simulink model "QPSK_Rayleigh_Channel"  (R2023b)
settings: Solver=FixedStepDiscrete  StartTime=0.0  StopTime=0.2  RelTol=1e-3  EnableMultiTasking=on
PreLoadFcn:
  | bitRate = 500000;
  | bitsPerFrame = 200;
  | maxDopplerShift = 200;
  | delayVector = [0:3]*(4e-6);
  | gainVector = [0:3]*(-3);
  | LOSDopplerShift = 100;
  | KFactor = 10;
undefined symbols (not defined in the file or in its folder): doppler
libraries: commchan3 x2, commrandsrc2 x1, commutil2 x1, commdigbbndam3 x1
CloseFcn:
  | clear bitRate
  | clear bitsPerFrame
  | clear maxDopplerShift
  | clear delayVector
  | clear gainVector
  | clear LOSDopplerShift
  | clear KFactor
Description:
  | Multipath Fading Channel
  | 
  | To learn about this model, click <a href="matlab: showdemo multipathfading_demo;">here</a>.
settings Model: Creator=The MathWorks Inc.  LastModifiedBy=Administrator
settings SolverCC: AlgebraicLoopSolver=TrustRegion
settings DataIOCC: SaveFormat=Array  SignalLoggingSaveFormat=ModelDataLogs  SaveOutput=off  SignalLogging=off  SaveTime=off  ReturnWorkspaceOutputs=off  SignalLoggingName=multipathSigsOut
settings OptimizationCC: BooleanDataType=off  OptimizeBlockIOStorage=off  BufferReuse=off  GlobalBufferReuse=off  ExpressionFolding=off  ExpressionDepthLimit=2147483647  LocalBlockOutputs=off  InitFltsAndDblsToZero=on  LifeSpan=inf  BufferReusableBoundary=off  OptimizeDataStoreBuffers=off  BusAssignmentInplaceUpdate=off
settings DebuggingCC: SaveWithParameterizedLinksMsg=none  UnderspecifiedInitializationDetection=Classic  MergeDetectMultiDrivingBlocksExec=none  CheckExecutionContextPreStartOutputMsg=on  SignalResolutionControl=TryResolveAllWithWarning  InheritedTsInSrcMsg=none  MultiTaskDSMMsg=warning  MultiTaskCondExecSysMsg=none  SigSpecEnsureSampleTimeMsg=none  FcnCallInpInsideContextMsg=warning  UnconnectedInputMsg=warning  UnconnectedOutputMsg=warning  UnconnectedLineMsg=warning  BusObjectLabelMismatch=none  StateNameClashWarn=warning  SFUnexpectedBacktrackingDiag=warning  SFNoUnconditionalDefaultTransitionDiag=warning  SFExecutionAtInitializationDiag=none  ArithmeticOperatorsInVariantConditions=warning
settings HardwareCC: ProdBitPerPointer=32  ProdBitPerSizeT=32  ProdBitPerPtrDiffT=32  ProdLargestAtomicFloat=None  ProdIntDivRoundTo=Undefined  ProdEndianess=Unspecified  ProdWordSize=32  ProdHWDeviceType=32-bit Generic  TargetUnknown=on
settings ModelReferenceCC: UpdateModelReferenceTargets=IfOutOfDate  EnableRefExpFcnMdlSchedulingChecks=on  PropagateSignalLabelsOutOfModel=off
settings SFSimCC: SimUseLocalCustomCode=off  CustomCodeUndefinedFunction=UseInterfaceOnly
settings RTWCC: RTWUseLocalCustomCode=off
settings CodeAppCC: StateflowObjectComments=on
settings GRTTargetCC: TargetFcnLib=ansi_tfl_tmw.mat  TargetLangStandard=C89/C90 (ANSI)  CombineOutputUpdateFcns=off  GRTInterface=on
settings ConfigComp: CovMetricSettings=dw  CovSaveCumulativeToWorkspaceVar=on  CovSaveSingleToWorkspaceVar=on  CovExternalEMLEnable=off

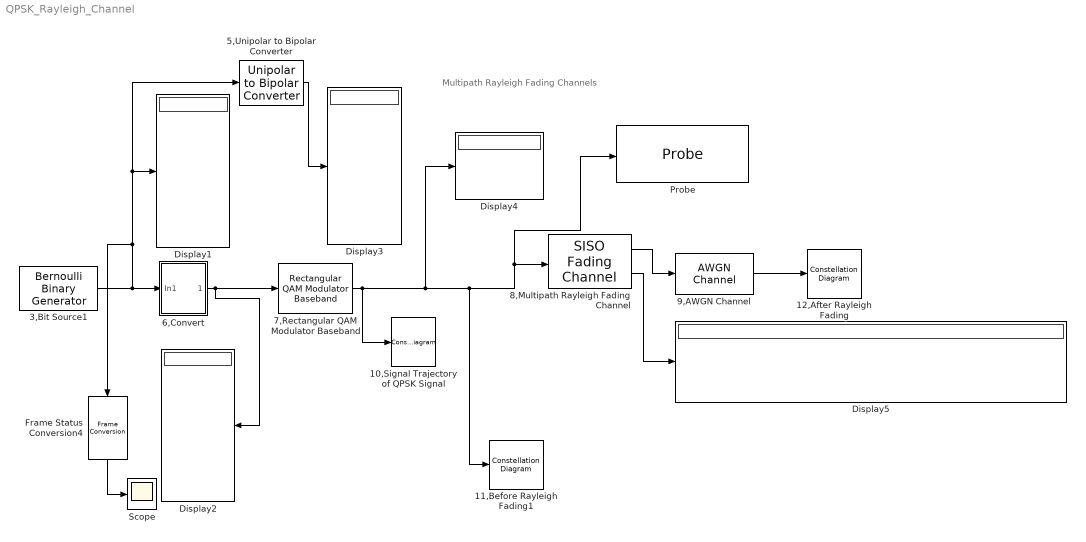
== system QPSK_Rayleigh_Channel ==
  note: Multipath Rayleigh Fading Channels
  10,Signal Trajectory of QPSK Signal : ConstellationDiagram  Tag=SignalTrajectory  WindowPosition=[297.000000,168.000000,490.000000,405.000000,]  ScopeFrameLocation=window  SymbolsToDisplaySource=Property  SymbolsToDisplay=1000  Title=Signal Trajectory of Noisy GMSK Signal  XLimits=[-1.25 1.25]  YLimits=[-1.25 1.25]  ShowTrajectory=on  ShowReferenceConstellation=off  ColorFading=on  DefaultConfigurationName=comm.scopes.ConstellationDiagramBlockCfg
      settings: OpenAtSimulationStart=off
  11,Before Rayleigh Fading1 : ConstellationDiagram  Tag=ScatterPlot  WindowPosition=[402.000000,174.000000,367.000000,395.000000,]  ScopeFrameLocation=window  SymbolsToDisplaySource=Property  SymbolsToDisplay=100  Title=Received signal after Rayleigh fading  XLimits=[-3.3 3.315]  YLimits=[-3.3 3.315]  ShowReferenceConstellation=off  ColorFading=on  DefaultConfigurationName=comm.scopes.ConstellationDiagramBlockCfg
      settings: OpenAtSimulationStart=off
  12,After Rayleigh Fading : ConstellationDiagram  Tag=ScatterPlot  WindowPosition=[15.000000,346.000000,346.000000,346.000000,]  Visible=on  ScopeFrameLocation=window  SymbolsToDisplaySource=Property  SymbolsToDisplay=100  Title=Received signal after Rayleigh fading  XLimits=[-1.3 1.3]  YLimits=[-1.3 1.3]  ShowReferenceConstellation=off  ColorFading=on  DefaultConfigurationName=comm.scopes.ConstellationDiagramBlockCfg
      settings: OpenAtSimulationStart=off
  3,Bit Source1 : commrandsrc2/Bernoulli Binary Generator  P=0.5  seed=61  Ts=1/500000  frameBased=on  sampPerFrame=8  orient=off  outDataType=double
  5,Unipolar to Bipolar Converter : commutil2/Unipolar to Bipolar Converter  M=2  polarity=Negative  dataType=Inherit via internal rule
  6,Convert : Subsystem
      mask Display: disp('convert')
  7,Rectangular QAM Modulator Baseband : commdigbbndam3/Rectangular QAM Modulator Baseband  M=4  InType=Bit  Enc=Gray  Mapping=[0,1,2,3]  PowType=Average Power  MinDist=2  AvgPow=1  PeakPow=1  Ph=-pi/2  outDtype=double  outWordLen=16  outUDDataType=sfix(16)  outFracLenMode=Best precision  outFracLen=15  outDataTypeStr=double  outLastDataTypeStr=double
  8,Multipath Rayleigh Fading Channel : commchan3/SISO Fading Channel  InheritSampleRate=off  SampleRate=250000  PathDelays=[0, 3, 8] .*1e-5  AveragePathGains=[0,-3,-6]  NormalizePathGains=on  FadingDistribution=Rayleigh  KFactor=3  DirectPathDopplerShift=0  DirectPathInitialPhase=0  MaximumDopplerShift=200  DopplerSpectrum=doppler('Jakes')  RandomStream=mt19937ar with seed  Seed=12345  PathGainsOutputPort=on  ChannelFilterDelayOutputPort=off  SimulateUsing=Interpreted execution  Visualization=Impulse response  PathsForDopplerDisplay=2  SamplesToDisplay=100%
  9,AWGN Channel : commchan3/AWGN Channel  LegacyMode=on  NoiseMethod="Signal to noise ratio  (SNR)"  noiseMode="Signal to noise ratio  (SNR)"  EbNo=10  EsNo=15  SNR=200  BitsPerSymbol=1  SignalPower=1  SamplesPerSymbol=1  SymbolPeriod=1e-6  VarianceSource=Parameter  Variance=1  RandomStream=Global stream  Seed=67  SimulateUsing=Code generation
  Display{1..5} (5 alike) : Display
  Frame Status Conversion4 : FrameConversion  OutFrame=Sample-based
  Probe : Probe  ProbeSignalDimensions=on
  Scope : Scope
  wires:
  9,AWGN Channel/1 -> 12,After Rayleigh Fading/1
  5,Unipolar to Bipolar Converter/1 -> Display3/1
  6,Convert/1(Out1) -> 7,Rectangular QAM Modulator Baseband/1, Display2/1
  3,Bit Source1/1 -> 6,Convert/1(In1), Display1/1, 5,Unipolar to Bipolar Converter/1, Frame Status Conversion4/1
  8,Multipath Rayleigh Fading Channel/1 -> 9,AWGN Channel/1
  Frame Status Conversion4/1 -> Scope/1
  7,Rectangular QAM Modulator Baseband/1 -> Display4/1, Probe/1, 8,Multipath Rayleigh Fading Channel/1, 11,Before Rayleigh Fading1/1, 10,Signal Trajectory of QPSK Signal/1
  8,Multipath Rayleigh Fading Channel/2 -> Display5/1

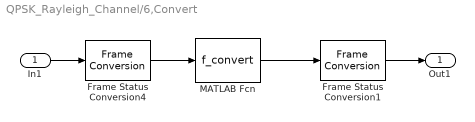
== system QPSK_Rayleigh_Channel/6,Convert ==
  In1 : Inport
  Frame Status Conversion1 : FrameConversion
  Frame Status Conversion4 : FrameConversion  OutFrame=Sample-based
  MATLAB Fcn : MATLABFcn  MATLABFcn=f_convert
  Out1 : Outport
  wires:
  MATLAB Fcn/1 -> Frame Status Conversion1/1
  Frame Status Conversion4/1 -> MATLAB Fcn/1
  In1/1 -> Frame Status Conversion4/1
  Frame Status Conversion1/1 -> Out1/1
